simulink model "nonlinear_model"  (R2016a)
settings: Solver=VariableStepAuto  StartTime=0.0  StopTime=T  MaxStep=1e-3  RelTol=1e-3
values from neighbouring files (symbols this model uses):
  a = 0.025    [constants.m]
  A = [ 0     0     0     0     1     0     0     0 ... (first row only)    [reduced_state_space.m]
  angular_velocity_0 = [0 0 0]    [simulation.m]
  B = [0 0 0 0 b_11 0    0    b_51 ... (first row only)    [reduced_state_space.m]
  C = [c_11 0    0    c_15 0 0 0 0 ... (first row only)    [reduced_state_space.m]
  g = 9.81305    [constants.m]
  h = 0.0095    [constants.m]
  I = [I_1  0    0 ... (first row only)    [constants.m]
  K = lqr(A, B, Q, R)    [reduced_state_space.m]
  Kr = (lqr(A',C',Q_r,R_r))'    [reduced_state_space.m]
  Ks = pocet_zavitu * prumerna_area    (= 0.0603185789489)    [constants.m]
  m = pi*r^2*h*neodymium_density    (= 0.0694645405617)    [constants.m]
  m_0 = 3.3906    [constants.m]
  m_2 = 1.5321    [constants.m]
  max_I = 2    [constants.m]
  noise_power = 1*10^(-11)    (= 1e-11)    [constants.m]
  perm_vak_4pi = 10^(-7)    (= 1e-07)    [constants.m]
  phi_0 = [0.00 0.00 0]    [simulation.m]
  R = [1 0 ... (first row only)    [reduced_state_space.m]
  rot_damp = 0*0.00002    (= 0)    [constants.m]
  s = 1*0.001    (= 0.001)    [constants.m]
  sample_period = 0.003    [constants.m]
  setpoint_x = perm_vak_4pi*m_0 * ( (3*s*z_r)/(s^2+z_r^2)^(5/2) )    [simulation.m]
  setpoint_y = setpoint_x    [simulation.m]
  x_0 = [0.001 -0.0015 z_r-0.000]    [simulation.m]
  x_1 = [-a  a 0]    [constants.m]
  x_2 = [ a  a 0]    [constants.m]
  x_3 = [-a -a 0]    [constants.m]
  x_4 = [ a -a 0]    [constants.m]
  x_5 = [ 0  a 0]    [constants.m]
  x_6 = [-a  0 0]    [constants.m]
  x_7 = [ a  0 0]    [constants.m]
  x_8 = [ 0 -a 0]    [constants.m]
undefined symbols (not defined in the file or in its folder): Kd, Ki, Kp, X, Y, Z
libraries: sm_lib x27, nesl_utility x9, simulink x8, vrlib x1
(part 1 of 2)
settings Model: Creator=tomas  LastModifiedBy=tomas
settings GRTTargetCC: GeneratePreprocessorConditionals=Use local settings
settings ExplorerConfigSet: InternalSimMechanicsExplorerSettings="<ExplorerConfiguration><canonicalview>default</canonicalview><AnimationSetting><BasePlaybackSpeed>1.0</BasePlaybackSpeed><PlaybackSpeedFactor>1.0</PlaybackSpeedFactor></AnimationSetting><TilePanel><TileInfo><Tiles Columns=\"1\" Count=\"1\" Rows=\"1\"><Column Left=\"2\" Weight=\"1\"/><Column Left=\"1556\"/><Row Top=\"2\" Weight=\"1\"/><Row Top=\"911\"/><Tile Height=\"1\" Width=\"1\" X=\"0\" Y=\"0\"/></Tiles></TileInfo><SceneInfo><SceneViewer><BGColor><R>0.60000002384185791</R><G>0.60000002384185791</G><B>0.60000002384185791</B></BGColor><Camera><DoPerspective>on</DoPerspective><Position><X>0.086098520718741134</X><Y>-0.08774684025324489</Y><Z>0.063402601032515923</Z></Position><Center><X>-0.0038966663563407573</X><Y>0.0036212337751197724</Y><Z>-0.0027823330820347203</Z></Center><Up><X>-0.3343595100680733</X><Y>0.314274704787183</Y><Z>0.88850161955843809</Z></Up><ViewLimDist>1</ViewLimDist><YLim>0.46630765815499858</YLim><XLim>0.80049481316608084</XLim></Camera></SceneViewer></SceneInfo></TilePanel><MechEditorPanel><Cameras><Camera><Id>Camera1</Id><Value><Name>Camera1</Name><NativeCamera><PositionKeyframeSet/><CenterKeyframeSet/><UpVectorKeyframeSet/></NativeCamera></Value></Camera></Cameras><GfxPanelCameraMap><MapElement CameraMLId=\"Camera1\" GfxPanelIndex=\"0\"/></GfxPanelCameraMap></MechEditorPanel></ExplorerConfiguration>"

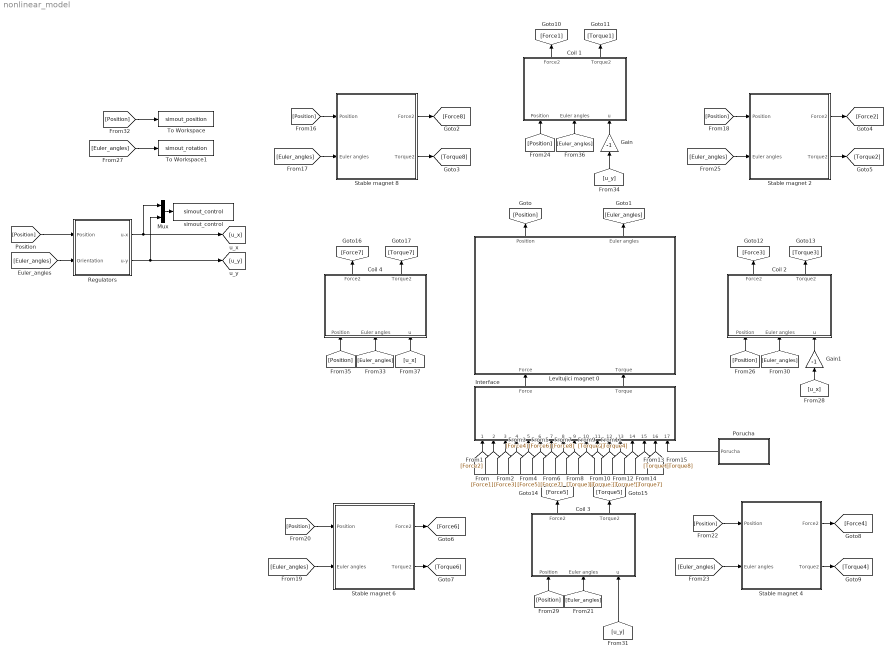
== system nonlinear_model ==
  Coil 1 : Subsystem
      mask Display: image(imread('obrazky/coil.jpg'))
  Coil 2 : Subsystem
      mask Display: image(imread('obrazky/coil.jpg'))
  Coil 3 : Subsystem
      mask Display: image(imread('obrazky/coil.jpg'))
  Coil 4 : Subsystem
      mask Display: image(imread('obrazky/coil.jpg'))
  Gain : Gain  Gain=-1
  Gain1 : Gain  Gain=-1
  Interface : Subsystem
      mask Display: image(imread('obrazky/interface.jpg'))
  Levitujici magnet 0 : Subsystem
      mask Display: image(imread('obrazky/levit.jpg'))
  Mux : Mux  Inputs=2
  Porucha : Subsystem
  Regulators : Subsystem
  Stable magnet 2 : Subsystem
      mask Display: image(imread('obrazky/stable.jpg'))
  Stable magnet 4 : Subsystem
      mask Display: image(imread('obrazky/stable.jpg'))
  Stable magnet 6 : Subsystem
      mask Display: image(imread('obrazky/stable.jpg'))
  Stable magnet 8 : Subsystem
      mask Display: image(imread('obrazky/stable.jpg'))
  To Workspace : ToWorkspace  VariableName=simout_position  SaveFormat=Timeseries  SampleTime=-1
  To Workspace1 : ToWorkspace  VariableName=simout_rotation  SaveFormat=Timeseries  SampleTime=-1
  simout_control : ToWorkspace  VariableName=simout_control  SaveFormat=Timeseries  SampleTime=-1
  wires:
  Levitujici magnet 0/1(Position) -> [Position]
  Levitujici magnet 0/2(Euler angles) -> [Euler_angles]
  [Force4] -> Interface/4(Force 4)
  [Force1] -> Interface/1(Force 1)
  [Force2] -> Interface/2(Force 2)
  [Force3] -> Interface/3(Force 3)
  [Force5] -> Interface/5(Force 5)
  [Force6] -> Interface/6(Force 6)
  [Force7] -> Interface/7(Force 7)
  [Force8] -> Interface/8(Force 8)
  [Torque1] -> Interface/9(Torque 1)
  [Torque2] -> Interface/10(Torque 2)
  [Torque3] -> Interface/11(Torque 3)
  [Torque4] -> Interface/12(Torque 4)
  [Torque5] -> Interface/13(Torque 5)
  [Torque6] -> Interface/14(Torque 6)
  [Torque7] -> Interface/15(Torque 7)
  [Torque8] -> Interface/16(Torque 8)
  Stable magnet 6/2(Torque2) -> [Torque6]
  [Euler_angles] -> Stable magnet 6/2(Euler angles)
  [Position] -> Stable magnet 6/1(Position)
  Stable magnet 6/1(Force2) -> [Force6]
  [Position] -> Coil 1/1(Position)
  [Euler_angles] -> Coil 1/2(Euler angles)
  Coil 1/1(Force2) -> [Force1]
  Coil 1/2(Torque2) -> [Torque1]
  Stable magnet 8/2(Torque2) -> [Torque8]
  [Euler_angles] -> Stable magnet 8/2(Euler angles)
  [Position] -> Stable magnet 8/1(Position)
  Stable magnet 8/1(Force2) -> [Force8]
  Stable magnet 2/2(Torque2) -> [Torque2]
  [Euler_angles] -> Stable magnet 2/2(Euler angles)
  [Position] -> Stable magnet 2/1(Position)
  Stable magnet 2/1(Force2) -> [Force2]
  [Position] -> To Workspace/1
  [Euler_angles] -> To Workspace1/1
  [u_y] -> Gain/1
  [Position] -> Coil 2/1(Position)
  [Euler_angles] -> Coil 2/2(Euler angles)
  Coil 2/1(Force2) -> [Force3]
  Coil 2/2(Torque2) -> [Torque3]
  [Position] -> Coil 3/1(Position)
  [Euler_angles] -> Coil 3/2(Euler angles)
  Coil 3/1(Force2) -> [Force5]
  Coil 3/2(Torque2) -> [Torque5]
  [Position] -> Coil 4/1(Position)
  [Euler_angles] -> Coil 4/2(Euler angles)
  Coil 4/1(Force2) -> [Force7]
  Coil 4/2(Torque2) -> [Torque7]
  [u_y] -> Coil 3/3(u)
  [u_x] -> Gain1/1
  [Position] -> Stable magnet 4/1(Position)
  [Euler_angles] -> Stable magnet 4/2(Euler angles)
  Stable magnet 4/1(Force2) -> [Force4]
  Stable magnet 4/2(Torque2) -> [Torque4]
  [u_x] -> Coil 4/3(u)
  Gain1/1 -> Coil 2/3(u)
  Interface/2(Torque) -> Levitujici magnet 0/2(Torque)
  Interface/1(Force) -> Levitujici magnet 0/1(Force)
  Gain/1 -> Coil 1/3(u)
  [Position] -> Regulators/1(Position)
  [Euler_angles] -> Regulators/2(Orientation)
  Mux/1 -> simout_control/1
  Regulators/2(u-y) -> [u_y], Mux/2
  Regulators/1(u-x) -> [u_x], Mux/1
  Porucha/1(Porucha) -> Interface/17(Porucha)

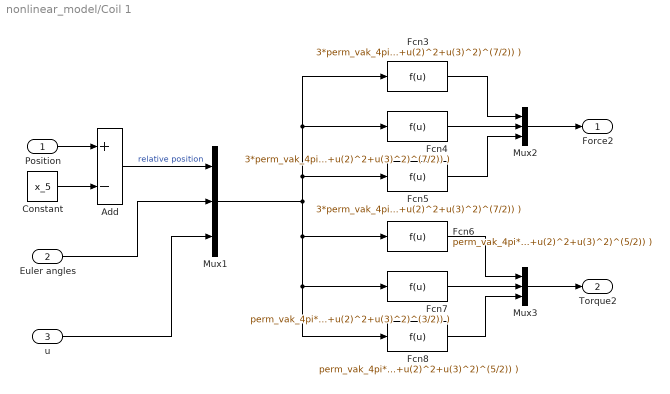
== system nonlinear_model/Coil 1 ==
  Position : Inport
  Euler angles : Inport  Port=2
  u : Inport  Port=3
  Add : Sum  Inputs=+-
  Constant : Constant  Value=x_5
  Fcn3 : Fcn  Expr=3*perm_vak_4pi*m_0*Ks*u(7) * ( (u(3)*(sin(u(4))*sin(u(6))+cos(u(4))*sin(u(5))*cos(u(6))))/((u(1)^2+u(2)^2+u(3)^2)^(5/2)) + (u(1)*(cos(u(4))*cos(u(5))))/((u(1)^2+u(2)^2+u(3)^2)^(5/2)) - (5*u(3)*u(1)*(u(1)*(sin(u(4))*sin(u(6))+cos(u(4))*sin(u(5))*cos(u(6)))+u(2)*(-sin(u(4))*cos(u(6))+cos(u(4))*sin(u(5))*sin(u(6)))+u(3)*(cos(u(4))*cos(u(5)))))/((u(1)^2+u(2)^2+u(3)^2)^(7/2)) )
  Fcn4 : Fcn  Expr=3*perm_vak_4pi*m_0*Ks*u(7) * ( (u(3)*(-sin(u(4))*cos(u(6))+cos(u(4))*sin(u(5))*sin(u(6))))/((u(1)^2+u(2)^2+u(3)^2)^(5/2)) + (u(2)*(cos(u(4))*cos(u(5))))/((u(1)^2+u(2)^2+u(3)^2)^(5/2)) - (5*u(3)*u(2)*(u(1)*(sin(u(4))*sin(u(6))+cos(u(4))*sin(u(5))*cos(u(6)))+u(2)*(-sin(u(4))*cos(u(6))+cos(u(4))*sin(u(5))*sin(u(6)))+u(3)*(cos(u(4))*cos(u(5)))))/((u(1)^2+u(2)^2+u(3)^2)^(7/2)) )
  Fcn5 : Fcn  Expr=3*perm_vak_4pi*m_0*Ks*u(7) * ( (u(3)*(cos(u(4))*cos(u(5))))/((u(1)^2+u(2)^2+u(3)^2)^(5/2)) + (u(1)*(sin(u(4))*sin(u(6))+cos(u(4))*sin(u(5))*cos(u(6)))+u(2)*(-sin(u(4))*cos(u(6))+cos(u(4))*sin(u(5))*sin(u(6)))+u(3)*(cos(u(4))*cos(u(5))))/((u(1)^2+u(2)^2+u(3)^2)^(5/2)) + (u(3)*(cos(u(4))*cos(u(5))))/((u(1)^2+u(2)^2+u(3)^2)^(5/2)) - (5*u(3)^2*(u(1)*(sin(u(4))*sin(u(6))+cos(u(4))*sin(u(5))*cos(u(6)))+u(2)*(-sin(u(4))*cos(u(6))+cos(u(4))*sin(u(5))*sin(u(6)))+u(3)*(cos(u(4))*cos(u(5)))))/((u(1)^2+u(2)^2+u(3)^2)^(7/2)) )
  Fcn6 : Fcn  Expr=perm_vak_4pi*m_0*Ks*u(7) * ( (3*u(3)^2*(-sin(u(4))*cos(u(6))+cos(u(4))*sin(u(5))*sin(u(6))))/((u(1)^2+u(2)^2+u(3)^2)^(5/2)) - ((-sin(u(4))*cos(u(6))+cos(u(4))*sin(u(5))*sin(u(6))))/((u(1)^2+u(2)^2+u(3)^2)^(3/2)) - (3*u(2)*u(3)*(cos(u(4))*cos(u(5))))/((u(1)^2+u(2)^2+u(3)^2)^(5/2)) )
  Fcn7 : Fcn  Expr=perm_vak_4pi*m_0*Ks*u(7) * ( (3*u(1)*u(3)*(cos(u(4))*cos(u(5))))/((u(1)^2+u(2)^2+u(3)^2)^(5/2)) - (3*u(3)^2*(sin(u(4))*sin(u(6))+cos(u(4))*sin(u(5))*cos(u(6))))/((u(1)^2+u(2)^2+u(3)^2)^(5/2)) + ((sin(u(4))*sin(u(6))+cos(u(4))*sin(u(5))*cos(u(6))))/((u(1)^2+u(2)^2+u(3)^2)^(3/2)) )
  Fcn8 : Fcn  Expr=perm_vak_4pi*m_0*Ks*u(7) * ( (3*u(2)*u(3)*(sin(u(4))*sin(u(6))+cos(u(4))*sin(u(5))*cos(u(6))))/((u(1)^2+u(2)^2+u(3)^2)^(5/2)) - (3*u(1)*u(3)*(-sin(u(4))*cos(u(6))+cos(u(4))*sin(u(5))*sin(u(6))))/((u(1)^2+u(2)^2+u(3)^2)^(5/2)) )
  Mux1 : Mux  Inputs=3
  Mux2 : Mux  Inputs=3
  Mux3 : Mux  Inputs=3
  Force2 : Outport
  Torque2 : Outport  Port=2
  wires:
  Position/1 -> Add/1
  Constant/1 -> Add/2
  Euler angles/1 -> Mux1/2
  Add/1 -> Mux1/1  "relative position"
  Mux1/1 -> Fcn6/1, Fcn7/1, Fcn8/1, Fcn4/1, Fcn3/1, Fcn5/1
  Fcn3/1 -> Mux2/1
  Fcn4/1 -> Mux2/2
  Fcn5/1 -> Mux2/3
  Fcn6/1 -> Mux3/1
  Fcn7/1 -> Mux3/2
  Fcn8/1 -> Mux3/3
  Mux2/1 -> Force2/1
  Mux3/1 -> Torque2/1
  u/1 -> Mux1/3

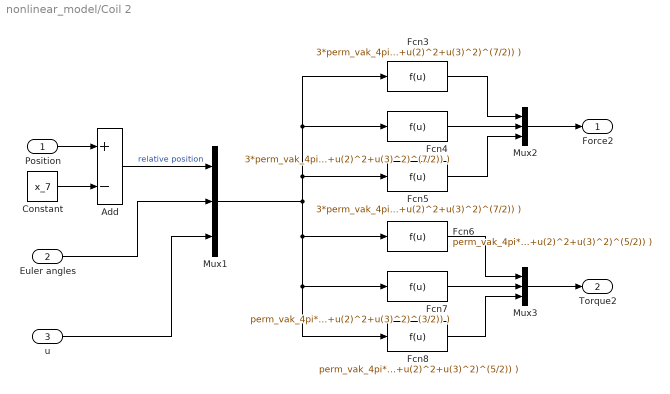
== system nonlinear_model/Coil 2 ==
  Position : Inport
  Euler angles : Inport  Port=2
  u : Inport  Port=3
  Add : Sum  Inputs=+-
  Constant : Constant  Value=x_7
  Fcn3 : Fcn  Expr=3*perm_vak_4pi*m_0*Ks*u(7) * ( (u(3)*(sin(u(4))*sin(u(6))+cos(u(4))*sin(u(5))*cos(u(6))))/((u(1)^2+u(2)^2+u(3)^2)^(5/2)) + (u(1)*(cos(u(4))*cos(u(5))))/((u(1)^2+u(2)^2+u(3)^2)^(5/2)) - (5*u(3)*u(1)*(u(1)*(sin(u(4))*sin(u(6))+cos(u(4))*sin(u(5))*cos(u(6)))+u(2)*(-sin(u(4))*cos(u(6))+cos(u(4))*sin(u(5))*sin(u(6)))+u(3)*(cos(u(4))*cos(u(5)))))/((u(1)^2+u(2)^2+u(3)^2)^(7/2)) )
  Fcn4 : Fcn  Expr=3*perm_vak_4pi*m_0*Ks*u(7) * ( (u(3)*(-sin(u(4))*cos(u(6))+cos(u(4))*sin(u(5))*sin(u(6))))/((u(1)^2+u(2)^2+u(3)^2)^(5/2)) + (u(2)*(cos(u(4))*cos(u(5))))/((u(1)^2+u(2)^2+u(3)^2)^(5/2)) - (5*u(3)*u(2)*(u(1)*(sin(u(4))*sin(u(6))+cos(u(4))*sin(u(5))*cos(u(6)))+u(2)*(-sin(u(4))*cos(u(6))+cos(u(4))*sin(u(5))*sin(u(6)))+u(3)*(cos(u(4))*cos(u(5)))))/((u(1)^2+u(2)^2+u(3)^2)^(7/2)) )
  Fcn5 : Fcn  Expr=3*perm_vak_4pi*m_0*Ks*u(7) * ( (u(3)*(cos(u(4))*cos(u(5))))/((u(1)^2+u(2)^2+u(3)^2)^(5/2)) + (u(1)*(sin(u(4))*sin(u(6))+cos(u(4))*sin(u(5))*cos(u(6)))+u(2)*(-sin(u(4))*cos(u(6))+cos(u(4))*sin(u(5))*sin(u(6)))+u(3)*(cos(u(4))*cos(u(5))))/((u(1)^2+u(2)^2+u(3)^2)^(5/2)) + (u(3)*(cos(u(4))*cos(u(5))))/((u(1)^2+u(2)^2+u(3)^2)^(5/2)) - (5*u(3)^2*(u(1)*(sin(u(4))*sin(u(6))+cos(u(4))*sin(u(5))*cos(u(6)))+u(2)*(-sin(u(4))*cos(u(6))+cos(u(4))*sin(u(5))*sin(u(6)))+u(3)*(cos(u(4))*cos(u(5)))))/((u(1)^2+u(2)^2+u(3)^2)^(7/2)) )
  Fcn6 : Fcn  Expr=perm_vak_4pi*m_0*Ks*u(7) * ( (3*u(3)^2*(-sin(u(4))*cos(u(6))+cos(u(4))*sin(u(5))*sin(u(6))))/((u(1)^2+u(2)^2+u(3)^2)^(5/2)) - ((-sin(u(4))*cos(u(6))+cos(u(4))*sin(u(5))*sin(u(6))))/((u(1)^2+u(2)^2+u(3)^2)^(3/2)) - (3*u(2)*u(3)*(cos(u(4))*cos(u(5))))/((u(1)^2+u(2)^2+u(3)^2)^(5/2)) )
  Fcn7 : Fcn  Expr=perm_vak_4pi*m_0*Ks*u(7) * ( (3*u(1)*u(3)*(cos(u(4))*cos(u(5))))/((u(1)^2+u(2)^2+u(3)^2)^(5/2)) - (3*u(3)^2*(sin(u(4))*sin(u(6))+cos(u(4))*sin(u(5))*cos(u(6))))/((u(1)^2+u(2)^2+u(3)^2)^(5/2)) + ((sin(u(4))*sin(u(6))+cos(u(4))*sin(u(5))*cos(u(6))))/((u(1)^2+u(2)^2+u(3)^2)^(3/2)) )
  Fcn8 : Fcn  Expr=perm_vak_4pi*m_0*Ks*u(7) * ( (3*u(2)*u(3)*(sin(u(4))*sin(u(6))+cos(u(4))*sin(u(5))*cos(u(6))))/((u(1)^2+u(2)^2+u(3)^2)^(5/2)) - (3*u(1)*u(3)*(-sin(u(4))*cos(u(6))+cos(u(4))*sin(u(5))*sin(u(6))))/((u(1)^2+u(2)^2+u(3)^2)^(5/2)) )
  Mux1 : Mux  Inputs=3
  Mux2 : Mux  Inputs=3
  Mux3 : Mux  Inputs=3
  Force2 : Outport
  Torque2 : Outport  Port=2
  wires:
  Position/1 -> Add/1
  Constant/1 -> Add/2
  Euler angles/1 -> Mux1/2
  Add/1 -> Mux1/1  "relative position"
  Mux1/1 -> Fcn6/1, Fcn7/1, Fcn8/1, Fcn4/1, Fcn3/1, Fcn5/1
  Fcn3/1 -> Mux2/1
  Fcn4/1 -> Mux2/2
  Fcn5/1 -> Mux2/3
  Fcn6/1 -> Mux3/1
  Fcn7/1 -> Mux3/2
  Fcn8/1 -> Mux3/3
  Mux2/1 -> Force2/1
  Mux3/1 -> Torque2/1
  u/1 -> Mux1/3

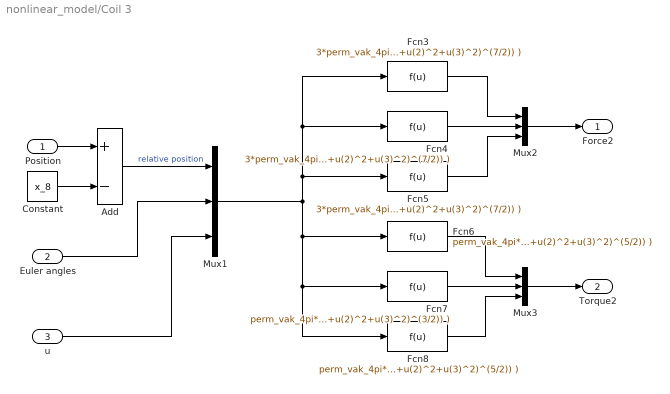
== system nonlinear_model/Coil 3 ==
  Position : Inport
  Euler angles : Inport  Port=2
  u : Inport  Port=3
  Add : Sum  Inputs=+-
  Constant : Constant  Value=x_8
  Fcn3 : Fcn  Expr=3*perm_vak_4pi*m_0*Ks*u(7) * ( (u(3)*(sin(u(4))*sin(u(6))+cos(u(4))*sin(u(5))*cos(u(6))))/((u(1)^2+u(2)^2+u(3)^2)^(5/2)) + (u(1)*(cos(u(4))*cos(u(5))))/((u(1)^2+u(2)^2+u(3)^2)^(5/2)) - (5*u(3)*u(1)*(u(1)*(sin(u(4))*sin(u(6))+cos(u(4))*sin(u(5))*cos(u(6)))+u(2)*(-sin(u(4))*cos(u(6))+cos(u(4))*sin(u(5))*sin(u(6)))+u(3)*(cos(u(4))*cos(u(5)))))/((u(1)^2+u(2)^2+u(3)^2)^(7/2)) )
  Fcn4 : Fcn  Expr=3*perm_vak_4pi*m_0*Ks*u(7) * ( (u(3)*(-sin(u(4))*cos(u(6))+cos(u(4))*sin(u(5))*sin(u(6))))/((u(1)^2+u(2)^2+u(3)^2)^(5/2)) + (u(2)*(cos(u(4))*cos(u(5))))/((u(1)^2+u(2)^2+u(3)^2)^(5/2)) - (5*u(3)*u(2)*(u(1)*(sin(u(4))*sin(u(6))+cos(u(4))*sin(u(5))*cos(u(6)))+u(2)*(-sin(u(4))*cos(u(6))+cos(u(4))*sin(u(5))*sin(u(6)))+u(3)*(cos(u(4))*cos(u(5)))))/((u(1)^2+u(2)^2+u(3)^2)^(7/2)) )
  Fcn5 : Fcn  Expr=3*perm_vak_4pi*m_0*Ks*u(7) * ( (u(3)*(cos(u(4))*cos(u(5))))/((u(1)^2+u(2)^2+u(3)^2)^(5/2)) + (u(1)*(sin(u(4))*sin(u(6))+cos(u(4))*sin(u(5))*cos(u(6)))+u(2)*(-sin(u(4))*cos(u(6))+cos(u(4))*sin(u(5))*sin(u(6)))+u(3)*(cos(u(4))*cos(u(5))))/((u(1)^2+u(2)^2+u(3)^2)^(5/2)) + (u(3)*(cos(u(4))*cos(u(5))))/((u(1)^2+u(2)^2+u(3)^2)^(5/2)) - (5*u(3)^2*(u(1)*(sin(u(4))*sin(u(6))+cos(u(4))*sin(u(5))*cos(u(6)))+u(2)*(-sin(u(4))*cos(u(6))+cos(u(4))*sin(u(5))*sin(u(6)))+u(3)*(cos(u(4))*cos(u(5)))))/((u(1)^2+u(2)^2+u(3)^2)^(7/2)) )
  Fcn6 : Fcn  Expr=perm_vak_4pi*m_0*Ks*u(7) * ( (3*u(3)^2*(-sin(u(4))*cos(u(6))+cos(u(4))*sin(u(5))*sin(u(6))))/((u(1)^2+u(2)^2+u(3)^2)^(5/2)) - ((-sin(u(4))*cos(u(6))+cos(u(4))*sin(u(5))*sin(u(6))))/((u(1)^2+u(2)^2+u(3)^2)^(3/2)) - (3*u(2)*u(3)*(cos(u(4))*cos(u(5))))/((u(1)^2+u(2)^2+u(3)^2)^(5/2)) )
  Fcn7 : Fcn  Expr=perm_vak_4pi*m_0*Ks*u(7) * ( (3*u(1)*u(3)*(cos(u(4))*cos(u(5))))/((u(1)^2+u(2)^2+u(3)^2)^(5/2)) - (3*u(3)^2*(sin(u(4))*sin(u(6))+cos(u(4))*sin(u(5))*cos(u(6))))/((u(1)^2+u(2)^2+u(3)^2)^(5/2)) + ((sin(u(4))*sin(u(6))+cos(u(4))*sin(u(5))*cos(u(6))))/((u(1)^2+u(2)^2+u(3)^2)^(3/2)) )
  Fcn8 : Fcn  Expr=perm_vak_4pi*m_0*Ks*u(7) * ( (3*u(2)*u(3)*(sin(u(4))*sin(u(6))+cos(u(4))*sin(u(5))*cos(u(6))))/((u(1)^2+u(2)^2+u(3)^2)^(5/2)) - (3*u(1)*u(3)*(-sin(u(4))*cos(u(6))+cos(u(4))*sin(u(5))*sin(u(6))))/((u(1)^2+u(2)^2+u(3)^2)^(5/2)) )
  Mux1 : Mux  Inputs=3
  Mux2 : Mux  Inputs=3
  Mux3 : Mux  Inputs=3
  Force2 : Outport
  Torque2 : Outport  Port=2
  wires:
  Position/1 -> Add/1
  Constant/1 -> Add/2
  Euler angles/1 -> Mux1/2
  Add/1 -> Mux1/1  "relative position"
  Mux1/1 -> Fcn6/1, Fcn7/1, Fcn8/1, Fcn4/1, Fcn3/1, Fcn5/1
  Fcn3/1 -> Mux2/1
  Fcn4/1 -> Mux2/2
  Fcn5/1 -> Mux2/3
  Fcn6/1 -> Mux3/1
  Fcn7/1 -> Mux3/2
  Fcn8/1 -> Mux3/3
  Mux2/1 -> Force2/1
  Mux3/1 -> Torque2/1
  u/1 -> Mux1/3

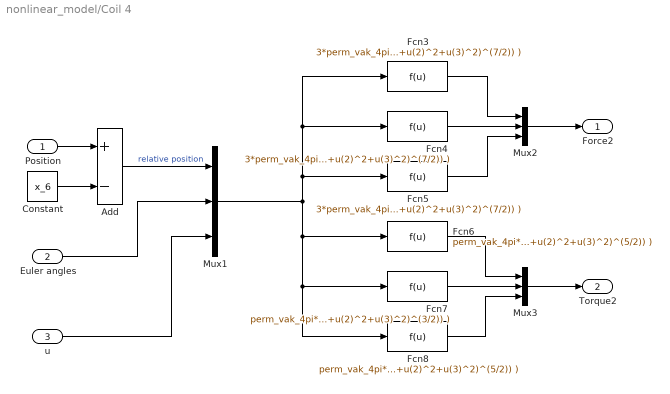
== system nonlinear_model/Coil 4 ==
  Position : Inport
  Euler angles : Inport  Port=2
  u : Inport  Port=3
  Add : Sum  Inputs=+-
  Constant : Constant  Value=x_6
  Fcn3 : Fcn  Expr=3*perm_vak_4pi*m_0*Ks*u(7) * ( (u(3)*(sin(u(4))*sin(u(6))+cos(u(4))*sin(u(5))*cos(u(6))))/((u(1)^2+u(2)^2+u(3)^2)^(5/2)) + (u(1)*(cos(u(4))*cos(u(5))))/((u(1)^2+u(2)^2+u(3)^2)^(5/2)) - (5*u(3)*u(1)*(u(1)*(sin(u(4))*sin(u(6))+cos(u(4))*sin(u(5))*cos(u(6)))+u(2)*(-sin(u(4))*cos(u(6))+cos(u(4))*sin(u(5))*sin(u(6)))+u(3)*(cos(u(4))*cos(u(5)))))/((u(1)^2+u(2)^2+u(3)^2)^(7/2)) )
  Fcn4 : Fcn  Expr=3*perm_vak_4pi*m_0*Ks*u(7) * ( (u(3)*(-sin(u(4))*cos(u(6))+cos(u(4))*sin(u(5))*sin(u(6))))/((u(1)^2+u(2)^2+u(3)^2)^(5/2)) + (u(2)*(cos(u(4))*cos(u(5))))/((u(1)^2+u(2)^2+u(3)^2)^(5/2)) - (5*u(3)*u(2)*(u(1)*(sin(u(4))*sin(u(6))+cos(u(4))*sin(u(5))*cos(u(6)))+u(2)*(-sin(u(4))*cos(u(6))+cos(u(4))*sin(u(5))*sin(u(6)))+u(3)*(cos(u(4))*cos(u(5)))))/((u(1)^2+u(2)^2+u(3)^2)^(7/2)) )
  Fcn5 : Fcn  Expr=3*perm_vak_4pi*m_0*Ks*u(7) * ( (u(3)*(cos(u(4))*cos(u(5))))/((u(1)^2+u(2)^2+u(3)^2)^(5/2)) + (u(1)*(sin(u(4))*sin(u(6))+cos(u(4))*sin(u(5))*cos(u(6)))+u(2)*(-sin(u(4))*cos(u(6))+cos(u(4))*sin(u(5))*sin(u(6)))+u(3)*(cos(u(4))*cos(u(5))))/((u(1)^2+u(2)^2+u(3)^2)^(5/2)) + (u(3)*(cos(u(4))*cos(u(5))))/((u(1)^2+u(2)^2+u(3)^2)^(5/2)) - (5*u(3)^2*(u(1)*(sin(u(4))*sin(u(6))+cos(u(4))*sin(u(5))*cos(u(6)))+u(2)*(-sin(u(4))*cos(u(6))+cos(u(4))*sin(u(5))*sin(u(6)))+u(3)*(cos(u(4))*cos(u(5)))))/((u(1)^2+u(2)^2+u(3)^2)^(7/2)) )
  Fcn6 : Fcn  Expr=perm_vak_4pi*m_0*Ks*u(7) * ( (3*u(3)^2*(-sin(u(4))*cos(u(6))+cos(u(4))*sin(u(5))*sin(u(6))))/((u(1)^2+u(2)^2+u(3)^2)^(5/2)) - ((-sin(u(4))*cos(u(6))+cos(u(4))*sin(u(5))*sin(u(6))))/((u(1)^2+u(2)^2+u(3)^2)^(3/2)) - (3*u(2)*u(3)*(cos(u(4))*cos(u(5))))/((u(1)^2+u(2)^2+u(3)^2)^(5/2)) )
  Fcn7 : Fcn  Expr=perm_vak_4pi*m_0*Ks*u(7) * ( (3*u(1)*u(3)*(cos(u(4))*cos(u(5))))/((u(1)^2+u(2)^2+u(3)^2)^(5/2)) - (3*u(3)^2*(sin(u(4))*sin(u(6))+cos(u(4))*sin(u(5))*cos(u(6))))/((u(1)^2+u(2)^2+u(3)^2)^(5/2)) + ((sin(u(4))*sin(u(6))+cos(u(4))*sin(u(5))*cos(u(6))))/((u(1)^2+u(2)^2+u(3)^2)^(3/2)) )
  Fcn8 : Fcn  Expr=perm_vak_4pi*m_0*Ks*u(7) * ( (3*u(2)*u(3)*(sin(u(4))*sin(u(6))+cos(u(4))*sin(u(5))*cos(u(6))))/((u(1)^2+u(2)^2+u(3)^2)^(5/2)) - (3*u(1)*u(3)*(-sin(u(4))*cos(u(6))+cos(u(4))*sin(u(5))*sin(u(6))))/((u(1)^2+u(2)^2+u(3)^2)^(5/2)) )
  Mux1 : Mux  Inputs=3
  Mux2 : Mux  Inputs=3
  Mux3 : Mux  Inputs=3
  Force2 : Outport
  Torque2 : Outport  Port=2
  wires:
  Position/1 -> Add/1
  Constant/1 -> Add/2
  Euler angles/1 -> Mux1/2
  Add/1 -> Mux1/1  "relative position"
  Mux1/1 -> Fcn6/1, Fcn7/1, Fcn8/1, Fcn4/1, Fcn3/1, Fcn5/1
  Fcn3/1 -> Mux2/1
  Fcn4/1 -> Mux2/2
  Fcn5/1 -> Mux2/3
  Fcn6/1 -> Mux3/1
  Fcn7/1 -> Mux3/2
  Fcn8/1 -> Mux3/3
  Mux2/1 -> Force2/1
  Mux3/1 -> Torque2/1
  u/1 -> Mux1/3

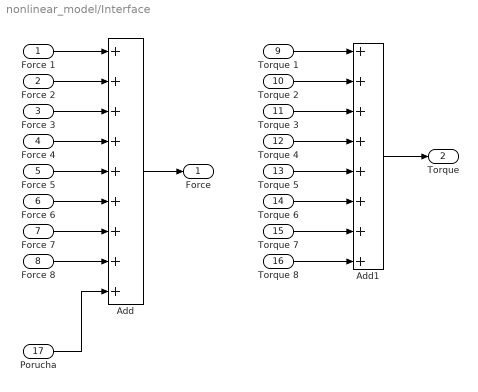
== system nonlinear_model/Interface ==
  Force 1 : Inport
  Force 2 : Inport  Port=2
  Force 3 : Inport  Port=3
  Force 4 : Inport  Port=4
  Force 5 : Inport  Port=5
  Force 6 : Inport  Port=6
  Force 7 : Inport  Port=7
  Force 8 : Inport  Port=8
  Torque 1 : Inport  Port=9
  Torque 2 : Inport  Port=10
  Torque 3 : Inport  Port=11
  Torque 4 : Inport  Port=12
  Torque 5 : Inport  Port=13
  Torque 6 : Inport  Port=14
  Torque 7 : Inport  Port=15
  Torque 8 : Inport  Port=16
  Porucha : Inport  Port=17
  Add : Sum  Inputs=9
  Add1 : Sum  Inputs=8
  Force : Outport
  Torque : Outport  Port=2
  wires:
  Force 1/1 -> Add/1
  Force 2/1 -> Add/2
  Force 3/1 -> Add/3
  Force 4/1 -> Add/4
  Force 5/1 -> Add/5
  Force 6/1 -> Add/6
  Force 7/1 -> Add/7
  Force 8/1 -> Add/8
  Add/1 -> Force/1
  Torque 8/1 -> Add1/8
  Torque 7/1 -> Add1/7
  Torque 6/1 -> Add1/6
  Torque 5/1 -> Add1/5
  Torque 4/1 -> Add1/4
  Torque 3/1 -> Add1/3
  Torque 2/1 -> Add1/2
  Torque 1/1 -> Add1/1
  Add1/1 -> Torque/1
  Porucha/1 -> Add/9

== system nonlinear_model/Levitujici magnet 0 ==
  Force : Inport
  Torque : Inport  Port=2
  Animation : Subsystem
  Constant : Constant  Commented=on  Value=x_0
  Constant1 : Constant  Commented=on  Value=[0 0 m*g]
  Force1 : InportShadow
  Orientation computation : Subsystem
  Position computation : Subsystem
  Position : Outport
  Euler angles : Outport  Port=2
  wires:
  Force/1 -> Position computation/1(Force)
  Orientation computation/1(Out1) -> Euler angles/1
  Position computation/1(Position) -> Position/1
  Force1/1 -> Animation/1(Force)
  Torque/1 -> Animation/2(Torque), Orientation computation/1(In1)

== system nonlinear_model/Porucha ==
  Add : Sum  Commented=on  Inputs=2
  Constant : Constant  Value=0
  Mux : Mux  Inputs=3
  Ramp : simulink/Sources/Ramp  Commented=on  slope=0.1  start=1  X0=0
  Sine Wave : Sin  Commented=on  Amplitude=0.03  Frequency=31*2  SampleTime=0
  Step : Step  Commented=on  After=0.06  SampleTime=0
  Step1 : Step  Commented=on  Time=1.01  After=-0.06  SampleTime=0
  Porucha : Outport
  wires:
  Step/1 -> Add/1
  Step1/1 -> Add/2
  Mux/1 -> Porucha/1
  Constant/1 -> Mux/1, Mux/2, Mux/3

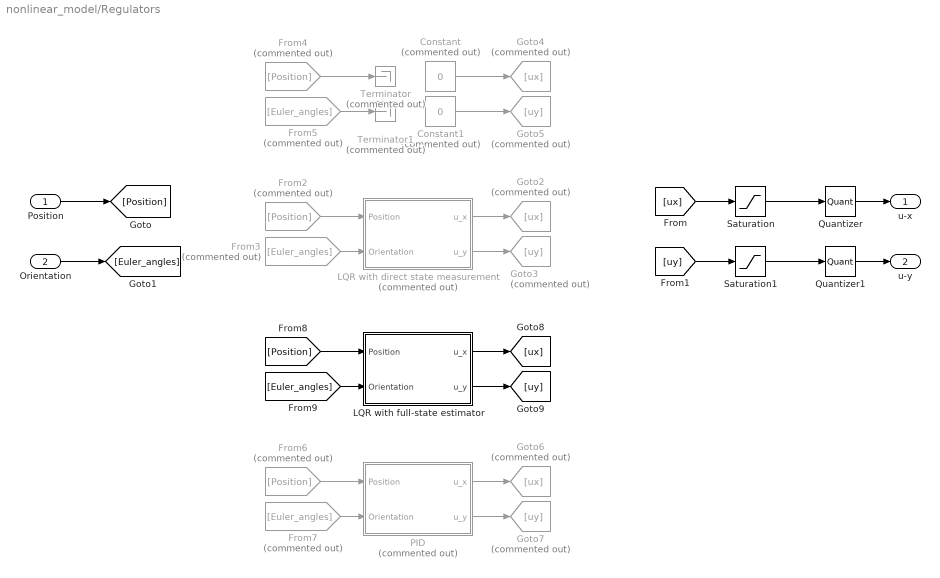
== system nonlinear_model/Regulators ==
  Position : Inport
  Orientation : Inport  Port=2
  Constant : Constant  Commented=on  Value=0
  Constant1 : Constant  Commented=on  Value=0
  From2 : From  Commented=on  GotoTag=Position
  From3 : From  Commented=on  GotoTag=Euler_angles
  From4 : From  Commented=on  GotoTag=Position
  From5 : From  Commented=on  GotoTag=Euler_angles
  From6 : From  Commented=on  GotoTag=Position
  From7 : From  Commented=on  GotoTag=Euler_angles
  Goto2 : Goto  Commented=on  GotoTag=ux
  Goto3 : Goto  Commented=on  GotoTag=uy
  Goto4 : Goto  Commented=on  GotoTag=ux
  Goto5 : Goto  Commented=on  GotoTag=uy
  Goto6 : Goto  Commented=on  GotoTag=ux
  Goto7 : Goto  Commented=on  GotoTag=uy
  LQR with direct state measurement : Subsystem  Commented=on
  LQR with full-state estimator : Subsystem
  PID : Subsystem  Commented=on
  Quantizer : Quantizer  QuantizationInterval=quantizer_konst
  Quantizer1 : Quantizer  QuantizationInterval=quantizer_konst
  Saturation : Saturate  UpperLimit=max_I  LowerLimit=-max_I
  Saturation1 : Saturate  UpperLimit=max_I  LowerLimit=-max_I
  Terminator : Terminator  Commented=on
  Terminator1 : Terminator  Commented=on
  u-x : Outport
  u-y : Outport  Port=2
  wires:
  Position/1 -> [Position]
  Orientation/1 -> [Euler_angles]
  From2/1 -> LQR with direct state measurement/1(Position)
  From3/1 -> LQR with direct state measurement/2(Orientation)
  LQR with direct state measurement/1(u_x) -> Goto2/1
  LQR with direct state measurement/2(u_y) -> Goto3/1
  [uy] -> Saturation1/1
  [ux] -> Saturation/1
  [Position] -> LQR with full-state estimator/1(Position)
  [Euler_angles] -> LQR with full-state estimator/2(Orientation)
  LQR with full-state estimator/1(u_x) -> [ux]
  LQR with full-state estimator/2(u_y) -> [uy]
  Quantizer/1 -> u-x/1
  Quantizer1/1 -> u-y/1
  From5/1 -> Terminator1/1
  From4/1 -> Terminator/1
  Constant1/1 -> Goto5/1
  Constant/1 -> Goto4/1
  From6/1 -> PID/1(Position)
  From7/1 -> PID/2(Orientation)
  PID/1(u_x) -> Goto6/1
  PID/2(u_y) -> Goto7/1
  Saturation/1 -> Quantizer/1
  Saturation1/1 -> Quantizer1/1

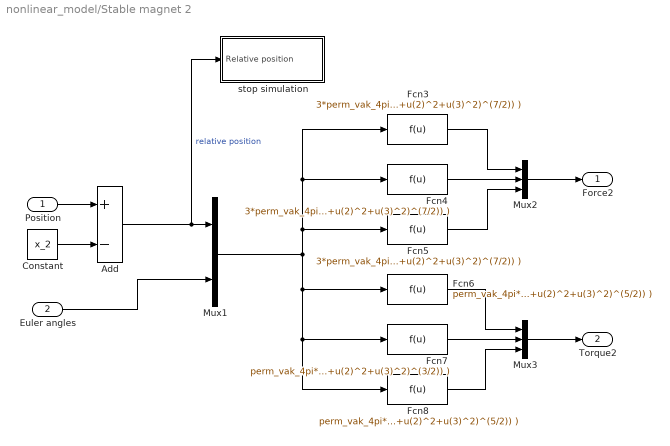
== system nonlinear_model/Stable magnet 2 ==
  Position : Inport
  Euler angles : Inport  Port=2
  Add : Sum  Inputs=+-
  Constant : Constant  Value=x_2
  Fcn3 : Fcn  Expr=3*perm_vak_4pi*m_2*m_0 * ( (u(3)*(sin(u(4))*sin(u(6))+cos(u(4))*sin(u(5))*cos(u(6))))/((u(1)^2+u(2)^2+u(3)^2)^(5/2)) + (u(1)*(cos(u(4))*cos(u(5))))/((u(1)^2+u(2)^2+u(3)^2)^(5/2)) - (5*u(3)*u(1)*(u(1)*(sin(u(4))*sin(u(6))+cos(u(4))*sin(u(5))*cos(u(6)))+u(2)*(-sin(u(4))*cos(u(6))+cos(u(4))*sin(u(5))*sin(u(6)))+u(3)*(cos(u(4))*cos(u(5)))))/((u(1)^2+u(2)^2+u(3)^2)^(7/2)) )
  Fcn4 : Fcn  Expr=3*perm_vak_4pi*m_2*m_0 * ( (u(3)*(-sin(u(4))*cos(u(6))+cos(u(4))*sin(u(5))*sin(u(6))))/((u(1)^2+u(2)^2+u(3)^2)^(5/2)) + (u(2)*(cos(u(4))*cos(u(5))))/((u(1)^2+u(2)^2+u(3)^2)^(5/2)) - (5*u(3)*u(2)*(u(1)*(sin(u(4))*sin(u(6))+cos(u(4))*sin(u(5))*cos(u(6)))+u(2)*(-sin(u(4))*cos(u(6))+cos(u(4))*sin(u(5))*sin(u(6)))+u(3)*(cos(u(4))*cos(u(5)))))/((u(1)^2+u(2)^2+u(3)^2)^(7/2)) )
  Fcn5 : Fcn  Expr=3*perm_vak_4pi*m_2*m_0 * ( (u(3)*(cos(u(4))*cos(u(5))))/((u(1)^2+u(2)^2+u(3)^2)^(5/2)) + (u(1)*(sin(u(4))*sin(u(6))+cos(u(4))*sin(u(5))*cos(u(6)))+u(2)*(-sin(u(4))*cos(u(6))+cos(u(4))*sin(u(5))*sin(u(6)))+u(3)*(cos(u(4))*cos(u(5))))/((u(1)^2+u(2)^2+u(3)^2)^(5/2)) + (u(3)*(cos(u(4))*cos(u(5))))/((u(1)^2+u(2)^2+u(3)^2)^(5/2)) - (5*u(3)^2*(u(1)*(sin(u(4))*sin(u(6))+cos(u(4))*sin(u(5))*cos(u(6)))+u(2)*(-sin(u(4))*cos(u(6))+cos(u(4))*sin(u(5))*sin(u(6)))+u(3)*(cos(u(4))*cos(u(5)))))/((u(1)^2+u(2)^2+u(3)^2)^(7/2)) )
  Fcn6 : Fcn  Expr=perm_vak_4pi*m_2*m_0 * ( (3*u(3)^2*(-sin(u(4))*cos(u(6))+cos(u(4))*sin(u(5))*sin(u(6))))/((u(1)^2+u(2)^2+u(3)^2)^(5/2)) - ((-sin(u(4))*cos(u(6))+cos(u(4))*sin(u(5))*sin(u(6))))/((u(1)^2+u(2)^2+u(3)^2)^(3/2)) - (3*u(2)*u(3)*(cos(u(4))*cos(u(5))))/((u(1)^2+u(2)^2+u(3)^2)^(5/2)) )
  Fcn7 : Fcn  Expr=perm_vak_4pi*m_2*m_0 * ( (3*u(1)*u(3)*(cos(u(4))*cos(u(5))))/((u(1)^2+u(2)^2+u(3)^2)^(5/2)) - (3*u(3)^2*(sin(u(4))*sin(u(6))+cos(u(4))*sin(u(5))*cos(u(6))))/((u(1)^2+u(2)^2+u(3)^2)^(5/2)) + ((sin(u(4))*sin(u(6))+cos(u(4))*sin(u(5))*cos(u(6))))/((u(1)^2+u(2)^2+u(3)^2)^(3/2)) )
  Fcn8 : Fcn  Expr=perm_vak_4pi*m_2*m_0 * ( (3*u(2)*u(3)*(sin(u(4))*sin(u(6))+cos(u(4))*sin(u(5))*cos(u(6))))/((u(1)^2+u(2)^2+u(3)^2)^(5/2)) - (3*u(1)*u(3)*(-sin(u(4))*cos(u(6))+cos(u(4))*sin(u(5))*sin(u(6))))/((u(1)^2+u(2)^2+u(3)^2)^(5/2)) )
  Mux1 : Mux  Inputs=2
  Mux2 : Mux  Inputs=3
  Mux3 : Mux  Inputs=3
  stop simulation : Subsystem
  Force2 : Outport
  Torque2 : Outport  Port=2
  wires:
  Position/1 -> Add/1
  Constant/1 -> Add/2
  Euler angles/1 -> Mux1/2
  Add/1 -> stop simulation/1("Relative position "), Mux1/1  "relative position"
  Mux1/1 -> Fcn6/1, Fcn7/1, Fcn8/1, Fcn4/1, Fcn3/1, Fcn5/1
  Fcn3/1 -> Mux2/1
  Fcn4/1 -> Mux2/2
  Fcn5/1 -> Mux2/3
  Fcn6/1 -> Mux3/1
  Fcn7/1 -> Mux3/2
  Fcn8/1 -> Mux3/3
  Mux2/1 -> Force2/1
  Mux3/1 -> Torque2/1

== system nonlinear_model/Stable magnet 4 ==
  Position : Inport
  Euler angles : Inport  Port=2
  Add : Sum  Inputs=+-
  Constant : Constant  Value=x_4
  Fcn3 : Fcn  Expr=3*perm_vak_4pi*m_2*m_0 * ( (u(3)*(sin(u(4))*sin(u(6))+cos(u(4))*sin(u(5))*cos(u(6))))/((u(1)^2+u(2)^2+u(3)^2)^(5/2)) + (u(1)*(cos(u(4))*cos(u(5))))/((u(1)^2+u(2)^2+u(3)^2)^(5/2)) - (5*u(3)*u(1)*(u(1)*(sin(u(4))*sin(u(6))+cos(u(4))*sin(u(5))*cos(u(6)))+u(2)*(-sin(u(4))*cos(u(6))+cos(u(4))*sin(u(5))*sin(u(6)))+u(3)*(cos(u(4))*cos(u(5)))))/((u(1)^2+u(2)^2+u(3)^2)^(7/2)) )
  Fcn4 : Fcn  Expr=3*perm_vak_4pi*m_2*m_0 * ( (u(3)*(-sin(u(4))*cos(u(6))+cos(u(4))*sin(u(5))*sin(u(6))))/((u(1)^2+u(2)^2+u(3)^2)^(5/2)) + (u(2)*(cos(u(4))*cos(u(5))))/((u(1)^2+u(2)^2+u(3)^2)^(5/2)) - (5*u(3)*u(2)*(u(1)*(sin(u(4))*sin(u(6))+cos(u(4))*sin(u(5))*cos(u(6)))+u(2)*(-sin(u(4))*cos(u(6))+cos(u(4))*sin(u(5))*sin(u(6)))+u(3)*(cos(u(4))*cos(u(5)))))/((u(1)^2+u(2)^2+u(3)^2)^(7/2)) )
  Fcn5 : Fcn  Expr=3*perm_vak_4pi*m_2*m_0 * ( (u(3)*(cos(u(4))*cos(u(5))))/((u(1)^2+u(2)^2+u(3)^2)^(5/2)) + (u(1)*(sin(u(4))*sin(u(6))+cos(u(4))*sin(u(5))*cos(u(6)))+u(2)*(-sin(u(4))*cos(u(6))+cos(u(4))*sin(u(5))*sin(u(6)))+u(3)*(cos(u(4))*cos(u(5))))/((u(1)^2+u(2)^2+u(3)^2)^(5/2)) + (u(3)*(cos(u(4))*cos(u(5))))/((u(1)^2+u(2)^2+u(3)^2)^(5/2)) - (5*u(3)^2*(u(1)*(sin(u(4))*sin(u(6))+cos(u(4))*sin(u(5))*cos(u(6)))+u(2)*(-sin(u(4))*cos(u(6))+cos(u(4))*sin(u(5))*sin(u(6)))+u(3)*(cos(u(4))*cos(u(5)))))/((u(1)^2+u(2)^2+u(3)^2)^(7/2)) )
  Fcn6 : Fcn  Expr=perm_vak_4pi*m_2*m_0 * ( (3*u(3)^2*(-sin(u(4))*cos(u(6))+cos(u(4))*sin(u(5))*sin(u(6))))/((u(1)^2+u(2)^2+u(3)^2)^(5/2)) - ((-sin(u(4))*cos(u(6))+cos(u(4))*sin(u(5))*sin(u(6))))/((u(1)^2+u(2)^2+u(3)^2)^(3/2)) - (3*u(2)*u(3)*(cos(u(4))*cos(u(5))))/((u(1)^2+u(2)^2+u(3)^2)^(5/2)) )
  Fcn7 : Fcn  Expr=perm_vak_4pi*m_2*m_0 * ( (3*u(1)*u(3)*(cos(u(4))*cos(u(5))))/((u(1)^2+u(2)^2+u(3)^2)^(5/2)) - (3*u(3)^2*(sin(u(4))*sin(u(6))+cos(u(4))*sin(u(5))*cos(u(6))))/((u(1)^2+u(2)^2+u(3)^2)^(5/2)) + ((sin(u(4))*sin(u(6))+cos(u(4))*sin(u(5))*cos(u(6))))/((u(1)^2+u(2)^2+u(3)^2)^(3/2)) )
  Fcn8 : Fcn  Expr=perm_vak_4pi*m_2*m_0 * ( (3*u(2)*u(3)*(sin(u(4))*sin(u(6))+cos(u(4))*sin(u(5))*cos(u(6))))/((u(1)^2+u(2)^2+u(3)^2)^(5/2)) - (3*u(1)*u(3)*(-sin(u(4))*cos(u(6))+cos(u(4))*sin(u(5))*sin(u(6))))/((u(1)^2+u(2)^2+u(3)^2)^(5/2)) )
  Mux1 : Mux  Inputs=2
  Mux2 : Mux  Inputs=3
  Mux3 : Mux  Inputs=3
  stop simulation : Subsystem
  Force2 : Outport
  Torque2 : Outport  Port=2
  wires:
  Position/1 -> Add/1
  Constant/1 -> Add/2
  Euler angles/1 -> Mux1/2
  Add/1 -> stop simulation/1("Relative position "), Mux1/1  "relative position"
  Mux1/1 -> Fcn6/1, Fcn7/1, Fcn8/1, Fcn4/1, Fcn3/1, Fcn5/1
  Fcn3/1 -> Mux2/1
  Fcn4/1 -> Mux2/2
  Fcn5/1 -> Mux2/3
  Fcn6/1 -> Mux3/1
  Fcn7/1 -> Mux3/2
  Fcn8/1 -> Mux3/3
  Mux2/1 -> Force2/1
  Mux3/1 -> Torque2/1

== system nonlinear_model/Stable magnet 6 ==
  Position : Inport
  Euler angles : Inport  Port=2
  Add : Sum  Inputs=+-
  Constant : Constant  Value=x_3
  Fcn3 : Fcn  Expr=3*perm_vak_4pi*m_2*m_0 * ( (u(3)*(sin(u(4))*sin(u(6))+cos(u(4))*sin(u(5))*cos(u(6))))/((u(1)^2+u(2)^2+u(3)^2)^(5/2)) + (u(1)*(cos(u(4))*cos(u(5))))/((u(1)^2+u(2)^2+u(3)^2)^(5/2)) - (5*u(3)*u(1)*(u(1)*(sin(u(4))*sin(u(6))+cos(u(4))*sin(u(5))*cos(u(6)))+u(2)*(-sin(u(4))*cos(u(6))+cos(u(4))*sin(u(5))*sin(u(6)))+u(3)*(cos(u(4))*cos(u(5)))))/((u(1)^2+u(2)^2+u(3)^2)^(7/2)) )
  Fcn4 : Fcn  Expr=3*perm_vak_4pi*m_2*m_0 * ( (u(3)*(-sin(u(4))*cos(u(6))+cos(u(4))*sin(u(5))*sin(u(6))))/((u(1)^2+u(2)^2+u(3)^2)^(5/2)) + (u(2)*(cos(u(4))*cos(u(5))))/((u(1)^2+u(2)^2+u(3)^2)^(5/2)) - (5*u(3)*u(2)*(u(1)*(sin(u(4))*sin(u(6))+cos(u(4))*sin(u(5))*cos(u(6)))+u(2)*(-sin(u(4))*cos(u(6))+cos(u(4))*sin(u(5))*sin(u(6)))+u(3)*(cos(u(4))*cos(u(5)))))/((u(1)^2+u(2)^2+u(3)^2)^(7/2)) )
  Fcn5 : Fcn  Expr=3*perm_vak_4pi*m_2*m_0 * ( (u(3)*(cos(u(4))*cos(u(5))))/((u(1)^2+u(2)^2+u(3)^2)^(5/2)) + (u(1)*(sin(u(4))*sin(u(6))+cos(u(4))*sin(u(5))*cos(u(6)))+u(2)*(-sin(u(4))*cos(u(6))+cos(u(4))*sin(u(5))*sin(u(6)))+u(3)*(cos(u(4))*cos(u(5))))/((u(1)^2+u(2)^2+u(3)^2)^(5/2)) + (u(3)*(cos(u(4))*cos(u(5))))/((u(1)^2+u(2)^2+u(3)^2)^(5/2)) - (5*u(3)^2*(u(1)*(sin(u(4))*sin(u(6))+cos(u(4))*sin(u(5))*cos(u(6)))+u(2)*(-sin(u(4))*cos(u(6))+cos(u(4))*sin(u(5))*sin(u(6)))+u(3)*(cos(u(4))*cos(u(5)))))/((u(1)^2+u(2)^2+u(3)^2)^(7/2)) )
  Fcn6 : Fcn  Expr=perm_vak_4pi*m_2*m_0 * ( (3*u(3)^2*(-sin(u(4))*cos(u(6))+cos(u(4))*sin(u(5))*sin(u(6))))/((u(1)^2+u(2)^2+u(3)^2)^(5/2)) - ((-sin(u(4))*cos(u(6))+cos(u(4))*sin(u(5))*sin(u(6))))/((u(1)^2+u(2)^2+u(3)^2)^(3/2)) - (3*u(2)*u(3)*(cos(u(4))*cos(u(5))))/((u(1)^2+u(2)^2+u(3)^2)^(5/2)) )
  Fcn7 : Fcn  Expr=perm_vak_4pi*m_2*m_0 * ( (3*u(1)*u(3)*(cos(u(4))*cos(u(5))))/((u(1)^2+u(2)^2+u(3)^2)^(5/2)) - (3*u(3)^2*(sin(u(4))*sin(u(6))+cos(u(4))*sin(u(5))*cos(u(6))))/((u(1)^2+u(2)^2+u(3)^2)^(5/2)) + ((sin(u(4))*sin(u(6))+cos(u(4))*sin(u(5))*cos(u(6))))/((u(1)^2+u(2)^2+u(3)^2)^(3/2)) )
  Fcn8 : Fcn  Expr=perm_vak_4pi*m_2*m_0 * ( (3*u(2)*u(3)*(sin(u(4))*sin(u(6))+cos(u(4))*sin(u(5))*cos(u(6))))/((u(1)^2+u(2)^2+u(3)^2)^(5/2)) - (3*u(1)*u(3)*(-sin(u(4))*cos(u(6))+cos(u(4))*sin(u(5))*sin(u(6))))/((u(1)^2+u(2)^2+u(3)^2)^(5/2)) )
  Mux1 : Mux  Inputs=2
  Mux2 : Mux  Inputs=3
  Mux3 : Mux  Inputs=3
  stop simulation : Subsystem
  Force2 : Outport
  Torque2 : Outport  Port=2
  wires:
  Position/1 -> Add/1
  Constant/1 -> Add/2
  Euler angles/1 -> Mux1/2
  Add/1 -> stop simulation/1("Relative position "), Mux1/1  "relative position"
  Mux1/1 -> Fcn6/1, Fcn7/1, Fcn8/1, Fcn4/1, Fcn3/1, Fcn5/1
  Fcn3/1 -> Mux2/1
  Fcn4/1 -> Mux2/2
  Fcn5/1 -> Mux2/3
  Fcn6/1 -> Mux3/1
  Fcn7/1 -> Mux3/2
  Fcn8/1 -> Mux3/3
  Mux2/1 -> Force2/1
  Mux3/1 -> Torque2/1

== system nonlinear_model/Stable magnet 8 ==
  Position : Inport
  Euler angles : Inport  Port=2
  Add : Sum  Inputs=+-
  Constant : Constant  Value=x_1
  Fcn3 : Fcn  Expr=3*perm_vak_4pi*m_2*m_0 * ( (u(3)*(sin(u(4))*sin(u(6))+cos(u(4))*sin(u(5))*cos(u(6))))/((u(1)^2+u(2)^2+u(3)^2)^(5/2)) + (u(1)*(cos(u(4))*cos(u(5))))/((u(1)^2+u(2)^2+u(3)^2)^(5/2)) - (5*u(3)*u(1)*(u(1)*(sin(u(4))*sin(u(6))+cos(u(4))*sin(u(5))*cos(u(6)))+u(2)*(-sin(u(4))*cos(u(6))+cos(u(4))*sin(u(5))*sin(u(6)))+u(3)*(cos(u(4))*cos(u(5)))))/((u(1)^2+u(2)^2+u(3)^2)^(7/2)) )
  Fcn4 : Fcn  Expr=3*perm_vak_4pi*m_2*m_0 * ( (u(3)*(-sin(u(4))*cos(u(6))+cos(u(4))*sin(u(5))*sin(u(6))))/((u(1)^2+u(2)^2+u(3)^2)^(5/2)) + (u(2)*(cos(u(4))*cos(u(5))))/((u(1)^2+u(2)^2+u(3)^2)^(5/2)) - (5*u(3)*u(2)*(u(1)*(sin(u(4))*sin(u(6))+cos(u(4))*sin(u(5))*cos(u(6)))+u(2)*(-sin(u(4))*cos(u(6))+cos(u(4))*sin(u(5))*sin(u(6)))+u(3)*(cos(u(4))*cos(u(5)))))/((u(1)^2+u(2)^2+u(3)^2)^(7/2)) )
  Fcn5 : Fcn  Expr=3*perm_vak_4pi*m_2*m_0 * ( (u(3)*(cos(u(4))*cos(u(5))))/((u(1)^2+u(2)^2+u(3)^2)^(5/2)) + (u(1)*(sin(u(4))*sin(u(6))+cos(u(4))*sin(u(5))*cos(u(6)))+u(2)*(-sin(u(4))*cos(u(6))+cos(u(4))*sin(u(5))*sin(u(6)))+u(3)*(cos(u(4))*cos(u(5))))/((u(1)^2+u(2)^2+u(3)^2)^(5/2)) + (u(3)*(cos(u(4))*cos(u(5))))/((u(1)^2+u(2)^2+u(3)^2)^(5/2)) - (5*u(3)^2*(u(1)*(sin(u(4))*sin(u(6))+cos(u(4))*sin(u(5))*cos(u(6)))+u(2)*(-sin(u(4))*cos(u(6))+cos(u(4))*sin(u(5))*sin(u(6)))+u(3)*(cos(u(4))*cos(u(5)))))/((u(1)^2+u(2)^2+u(3)^2)^(7/2)) )
  Fcn6 : Fcn  Expr=perm_vak_4pi*m_2*m_0 * ( (3*u(3)^2*(-sin(u(4))*cos(u(6))+cos(u(4))*sin(u(5))*sin(u(6))))/((u(1)^2+u(2)^2+u(3)^2)^(5/2)) - ((-sin(u(4))*cos(u(6))+cos(u(4))*sin(u(5))*sin(u(6))))/((u(1)^2+u(2)^2+u(3)^2)^(3/2)) - (3*u(2)*u(3)*(cos(u(4))*cos(u(5))))/((u(1)^2+u(2)^2+u(3)^2)^(5/2)) )
  Fcn7 : Fcn  Expr=perm_vak_4pi*m_2*m_0 * ( (3*u(1)*u(3)*(cos(u(4))*cos(u(5))))/((u(1)^2+u(2)^2+u(3)^2)^(5/2)) - (3*u(3)^2*(sin(u(4))*sin(u(6))+cos(u(4))*sin(u(5))*cos(u(6))))/((u(1)^2+u(2)^2+u(3)^2)^(5/2)) + ((sin(u(4))*sin(u(6))+cos(u(4))*sin(u(5))*cos(u(6))))/((u(1)^2+u(2)^2+u(3)^2)^(3/2)) )
  Fcn8 : Fcn  Expr=perm_vak_4pi*m_2*m_0 * ( (3*u(2)*u(3)*(sin(u(4))*sin(u(6))+cos(u(4))*sin(u(5))*cos(u(6))))/((u(1)^2+u(2)^2+u(3)^2)^(5/2)) - (3*u(1)*u(3)*(-sin(u(4))*cos(u(6))+cos(u(4))*sin(u(5))*sin(u(6))))/((u(1)^2+u(2)^2+u(3)^2)^(5/2)) )
  Mux1 : Mux  Inputs=2
  Mux2 : Mux  Inputs=3
  Mux3 : Mux  Inputs=3
  stop simulation : Subsystem
  Force2 : Outport
  Torque2 : Outport  Port=2
  wires:
  Position/1 -> Add/1
  Constant/1 -> Add/2
  Euler angles/1 -> Mux1/2
  Add/1 -> stop simulation/1("Relative position "), Mux1/1  "relative position"
  Mux1/1 -> Fcn6/1, Fcn7/1, Fcn8/1, Fcn4/1, Fcn3/1, Fcn5/1
  Fcn3/1 -> Mux2/1
  Fcn4/1 -> Mux2/2
  Fcn5/1 -> Mux2/3
  Fcn6/1 -> Mux3/1
  Fcn7/1 -> Mux3/2
  Fcn8/1 -> Mux3/3
  Mux2/1 -> Force2/1
  Mux3/1 -> Torque2/1
